simulink model "easy"  (Simulink 8.3)
settings: Solver=ode3  StartTime=0.0  StopTime=stop_time  FixedStep=step  RelTol=1e-3
values from neighbouring files (symbols this model uses):
  K = k_y/(k_e*i_p)    (= 0.649262481742)    [test_2.m]
  K_a = 10/alpha_max    (= 1.5888147442)    [test_2.m]
  K_f = R/(k_m*k_e*i_p^2)    (= 0.00467568734851)    [test_2.m]
  K_w = 10/w_0    (= 0.0770104563348)    [test_2.m]
  M_cm = 0    [test_2.m]
  T_m = R*J_sum/(k_m*k_e)    (= 0.0205730243334)    [test_2.m]
  U = 5    [test_2.m]
settings Model: Creator=Павел  LastModifiedBy=Павел
settings DataIOCC: SignalLoggingSaveFormat=Dataset
settings DebuggingCC: UnderspecifiedInitializationDetection=Simplified  StateNameClashWarn=none
settings GRTTargetCC: CombineOutputUpdateFcns=on  GRTInterface=off

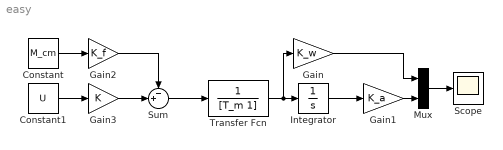
== system easy ==
  Constant : Constant  Value=M_cm
  Constant1 : Constant  Value=U
  Gain : Gain  Gain=K_w
  Gain1 : Gain  Gain=K_a
  Gain2 : Gain  Gain=K_f
  Gain3 : Gain  Gain=K
  Integrator : Integrator
  Mux : Mux  Inputs=2
  Scope : Scope
  Sum : Sum  Inputs=-+|
  Transfer Fcn : TransferFcn  Denominator=[T_m 1]
  wires:
  Mux/1 -> Scope/1
  Integrator/1 -> Gain1/1
  Transfer Fcn/1 -> Gain/1, Integrator/1
  Constant/1 -> Gain2/1
  Constant1/1 -> Gain3/1
  Gain/1 -> Mux/1
  Gain1/1 -> Mux/2
  Sum/1 -> Transfer Fcn/1
  Gain3/1 -> Sum/2
  Gain2/1 -> Sum/1
